simulink model "final_seatmodel2019a"  (R2019a)
settings: Solver=FixedStepAuto  StartTime=0.0  StopTime=50  FixedStep=1  RelTol=1e-3
libraries: powerlib_meascontrol x1
settings Model: Creator=A  LastModifiedBy=A

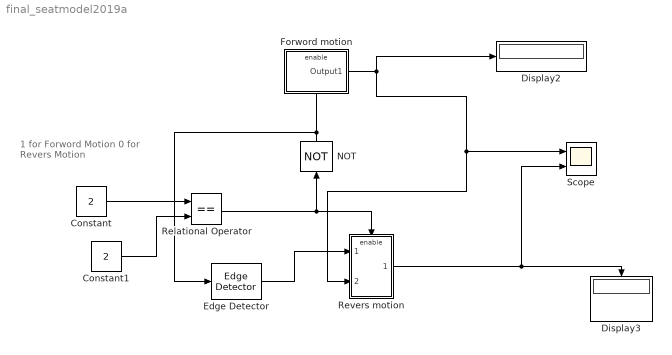
== system final_seatmodel2019a ==
  note: 1 for Forword Motion 0 for Revers Motion
  Constant : Constant  Value=2
  Constant1 : Constant  Value=2
  Display2 : Display
  Display3 : Display
  Edge Detector : powerlib_meascontrol/Logic/Edge Detector  model=Falling  ic=0  Ts=0
      settings: SourceProductBaseCode=PS
  Forword motion : Subsystem
  NOT : Logic  Operator=NOT  IconShape=distinctive  AllPortsSameDT=off  OutDataTypeStr=boolean
  Relational Operator : RelationalOperator  Operator===  OutDataTypeStr=boolean  RndMeth=Simplest
  Revers motion : Subsystem
  Scope : Scope  NumInputPorts=2
  wires:
  Relational Operator/1 -> Revers motion/Enable, NOT/1
  Constant/1 -> Relational Operator/1
  Forword motion/1(Output1) -> Display2/1, Revers motion/2(Input1), Scope/1
  Constant1/1 -> Relational Operator/2
  Revers motion/1(Output) -> Display3/1, Scope/2
  NOT/1 -> Edge Detector/1, Forword motion/Enable
  Edge Detector/1 -> Revers motion/1(Input)

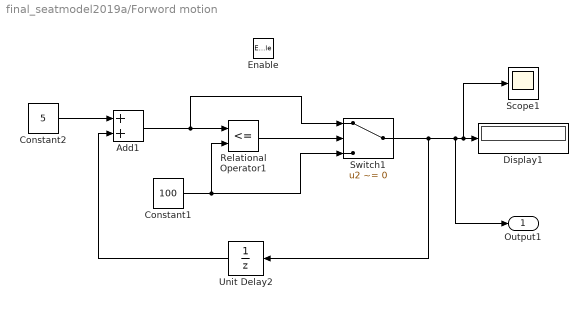
== system final_seatmodel2019a/Forword motion ==
  Enable : EnablePort
  Add1 : Sum
  Constant1 : Constant  Value=100
  Constant2 : Constant  Value=5
  Display1 : Display
  Relational Operator1 : RelationalOperator  Operator=<=  OutDataTypeStr=boolean  RndMeth=Simplest
  Scope1 : Scope
  Switch1 : Switch  Criteria=u2 ~= 0
  Unit Delay2 : UnitDelay  InitialCondition=-1  SampleTime=-1  HasFrameUpgradeWarning=on
  Output1 : Outport
  wires:
  Unit Delay2/1 -> Add1/2
  Constant1/1 -> Switch1/3, Relational Operator1/2
  Relational Operator1/1 -> Switch1/2
  Constant2/1 -> Add1/1
  Add1/1 -> Switch1/1, Relational Operator1/1
  Switch1/1 -> Unit Delay2/1, Output1/1, Scope1/1, Display1/1

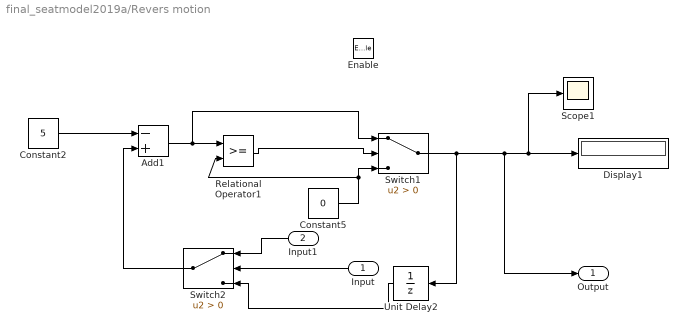
== system final_seatmodel2019a/Revers motion ==
  Input : Inport
  Input1 : Inport  Port=2
  Enable : EnablePort
  Add1 : Sum  Inputs=-+
  Constant2 : Constant  Value=5
  Constant5 : Constant  Value=0
  Display1 : Display
  Relational Operator1 : RelationalOperator  OutDataTypeStr=boolean  RndMeth=Simplest
  Scope1 : Scope
  Switch1 : Switch  Criteria=u2 > Threshold
  Switch2 : Switch  Criteria=u2 > Threshold
  Unit Delay2 : UnitDelay  InitialCondition=100  SampleTime=-1  HasFrameUpgradeWarning=on
  Output : Outport
  wires:
  Relational Operator1/1 -> Switch1/2
  Constant2/1 -> Add1/1
  Add1/1 -> Switch1/1, Relational Operator1/1
  Constant5/1 -> Relational Operator1/2, Switch1/3
  Switch1/1 -> Unit Delay2/1, Output/1, Display1/1, Scope1/1
  Switch2/1 -> Add1/2
  Input1/1 -> Switch2/1
  Unit Delay2/1 -> Switch2/3
  Input/1 -> Switch2/2
